simulink model "hw_ekf_est_all_para"  (R2021b)
settings: Solver=ode1  StartTime=0.0  StopTime=120  FixedStep=0.01  RelTol=1e-3  EnableMultiTasking=on
libraries: arduinolib x6, arduinosensorlib x1
settings Model: ExtModeTrigDuration=2  Creator=Admin  LastModifiedBy=ASUS
settings SolverCC: AlgebraicLoopSolver=TrustRegion  AutoInsertRateTranBlk=on
settings OptimizationCC: EnhancedBackFolding=on  PassReuseOutputArgsAs=Individual arguments  ZeroExternalMemoryAtStartup=off  ZeroInternalMemoryAtStartup=off  MaxStackSize=64  OptimizeBlockOrder=speed  DifferentSizesBufferReuse=on  OptimizationCustomize=off  EfficientTunableParamExpr=on
settings DebuggingCC: ParameterTunabilityLossMsg=error  SFMachineParentedDataDiag=warning
settings HardwareCC: ProdBitPerInt=16  ProdBitPerPointer=16  ProdBitPerSizeT=16  ProdBitPerPtrDiffT=16  ProdLargestAtomicFloat=None  ProdWordSize=8  ProdHWDeviceType=Atmel->AVR
settings SFSimCC: MATLABDynamicMemAlloc=off
settings RTWCC: Description=Embedded Coder  SystemTargetFile=ert.tlc  HardwareBoard=Arduino Mega 2560  TemplateMakefile=ert_default_tmf  Toolchain=Arduino AVR  BuildConfiguration=Faster Runs
settings CodeAppCC: ForceParamTrailComments=on  IgnoreCustomStorageClasses=off  OperatorAnnotations=on  SimulinkDataObjDesc=on  SFDataObjDesc=on  InsertBlockDesc=on
settings ERTTargetCC: SupportContinuousTime=on  SupportVariableSizeSignals=on  ExtModeTransport=3  ExtModeStaticAlloc=on  ExtModeStaticAllocSize=2048  ExtModeMexFile=ext_xcp  ExtModeIntrfLevel=Level2 - Open

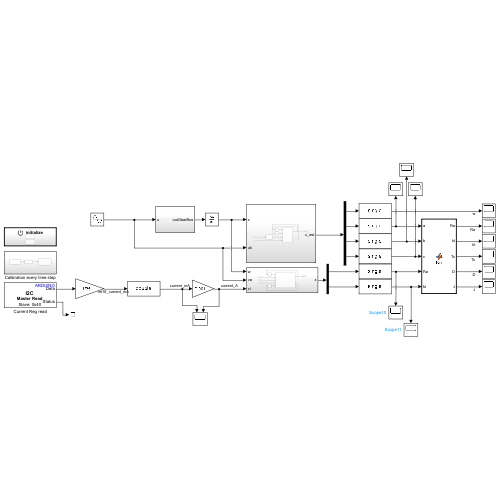
[thumbnail: Simulink's stored preview of the top-level diagram]
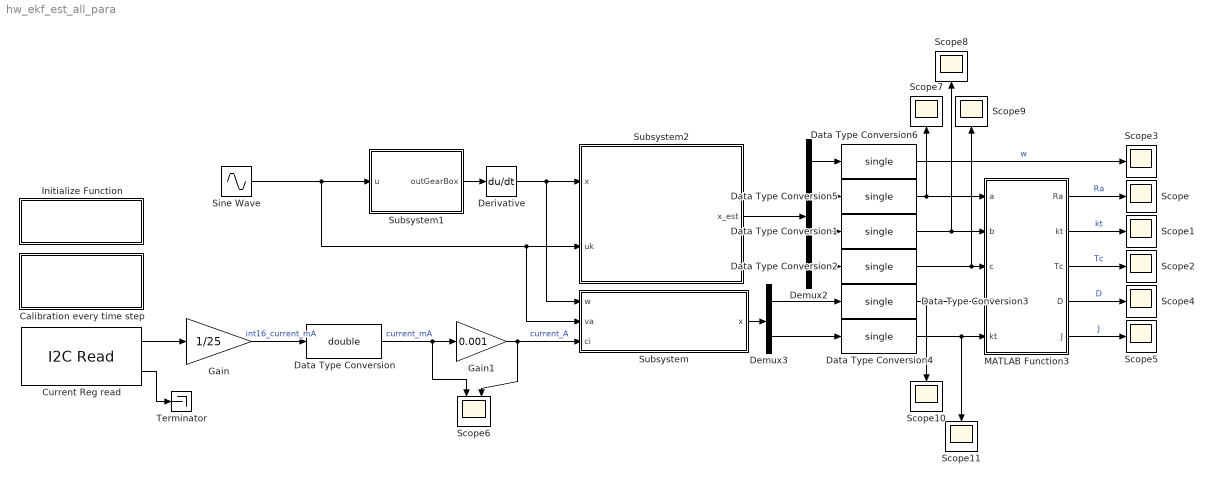
== system hw_ekf_est_all_para ==
  Calibration every time step : Subsystem  Priority=0
  Current Reg read : arduinolib/I2C Read  I2CModule=0  Mode=Master  SlaveAddress="hex2dec(\"0x40\")"  SlaveByteOrder=BigEndian  Direction=Receiver  RegisterAddressMode=on  RegisterAddress="hex2dec(\"0x04\")"  SlaveDataType=int16  DataLength=1  NoAck=off  RepeatedStart=off  OutputStatus=on  blockPlatform=ARDUINO  SampleTime=0.01
      settings: SourceProductBaseCode=ARDUINO
  Data Type Conversion : DataTypeConversion  OutDataTypeStr=double
  Data Type Conversion{1..6} (6 alike) : DataTypeConversion  OutDataTypeStr=single
  Demux2 : Demux
  Demux3 : Demux  Outputs=2
  Derivative : Derivative
  Gain : Gain  Gain=1/25
  Gain1 : Gain  Gain=0.001
  Initialize Function : Subsystem  TreatAsAtomicUnit=on
  MATLAB Function3 : MATLAB Function  TreatAsAtomicUnit=on
  Scope{,1..5,7..11} (11 alike) : Scope
  Scope6 : Scope  NumInputPorts=2
  Sine Wave : Sin  Amplitude=10  Frequency=2*pi*0.4  SampleTime=0
  Subsystem : Subsystem
  Subsystem1 : Subsystem
  Subsystem2 : Subsystem
  Terminator : Terminator
  wires:
  Demux3/2 -> Data Type Conversion4/1
  Demux2/4 -> Data Type Conversion2/1
  Demux2/3 -> Data Type Conversion1/1
  Subsystem2/1(x_est) -> Demux2/1
  Demux2/2 -> Data Type Conversion5/1
  Demux3/1 -> Data Type Conversion3/1
  Subsystem/1(x) -> Demux3/1
  Data Type Conversion/1 -> Scope6/1, Gain1/1  "current_mA"
  Current Reg read/2 -> Terminator/1
  Gain/1 -> Data Type Conversion/1  "int16_current_mA"
  Current Reg read/1 -> Gain/1
  Sine Wave/1 -> Subsystem1/1(u), Subsystem/2(va), Subsystem2/2(uk)
  Gain1/1 -> Subsystem/3(ci), Scope6/2  "current_A"
  Subsystem1/1(outGearBox) -> Derivative/1
  Derivative/1 -> Subsystem/1(w), Subsystem2/1(x)
  MATLAB Function3/1(Ra) -> Scope/1  "Ra"
  MATLAB Function3/2(kt) -> Scope1/1  "kt"
  MATLAB Function3/3(Tc) -> Scope2/1  "Tc"
  MATLAB Function3/4(D) -> Scope4/1  "D"
  MATLAB Function3/5(J) -> Scope5/1  "J"
  Demux2/1 -> Data Type Conversion6/1
  Data Type Conversion5/1 -> MATLAB Function3/1(a), Scope7/1
  Data Type Conversion1/1 -> Scope8/1, MATLAB Function3/2(b)
  Data Type Conversion2/1 -> Scope9/1, MATLAB Function3/3(c)
  Data Type Conversion3/1 -> Scope10/1, MATLAB Function3/4("Ra ")
  Data Type Conversion4/1 -> Scope11/1, MATLAB Function3/5("kt ")
  Data Type Conversion6/1 -> Scope3/1  "w"

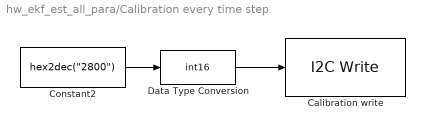
== system hw_ekf_est_all_para/Calibration every time step ==
  Calibration write : arduinolib/I2C Write  I2CModule=0  Mode=Master  SlaveAddress="uint8(hex2dec(\"0x40\"))"  SlaveByteOrder=BigEndian  Direction=Transmitter  RegisterAddressMode=on  RegisterAddress="uint8(hex2dec(\"0x05\"))"  SlaveDataType=uint8  DataLength=1  NoAck=off  RepeatedStart=off  OutputStatus=off  blockPlatform=ARDUINO
      settings: SourceProductBaseCode=ARDUINO
  Constant2 : Constant  Value="hex2dec(\"2800\")"
  Data Type Conversion : DataTypeConversion  OutDataTypeStr=int16
  wires:
  Constant2/1 -> Data Type Conversion/1
  Data Type Conversion/1 -> Calibration write/1

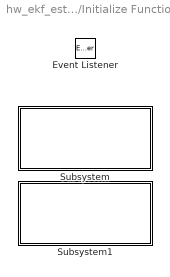
== system hw_ekf_est_all_para/Initialize Function ==
  Event Listener : EventListener  DisableCoverage=on  EventName=reset
  Subsystem : Subsystem  Priority=0
  Subsystem1 : Subsystem  Priority=1

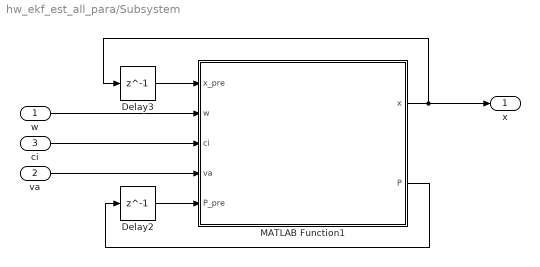
== system hw_ekf_est_all_para/Subsystem ==
  w : Inport
  va : Inport  Port=2
  ci : Inport  Port=3
  Delay2 : Delay  DelayLength=1  InitialCondition=diag([5,0.1])
  Delay3 : Delay  DelayLength=1  InitialCondition=[5;0.4]
  MATLAB Function1 : MATLAB Function  TreatAsAtomicUnit=on
  x : Outport
  wires:
  MATLAB Function1/1(x) -> x/1, Delay3/1
  Delay2/1 -> MATLAB Function1/5(P_pre)
  MATLAB Function1/2(P) -> Delay2/1
  Delay3/1 -> MATLAB Function1/1(x_pre)
  ci/1 -> MATLAB Function1/3(ci)
  w/1 -> MATLAB Function1/2(w)
  va/1 -> MATLAB Function1/4(va)

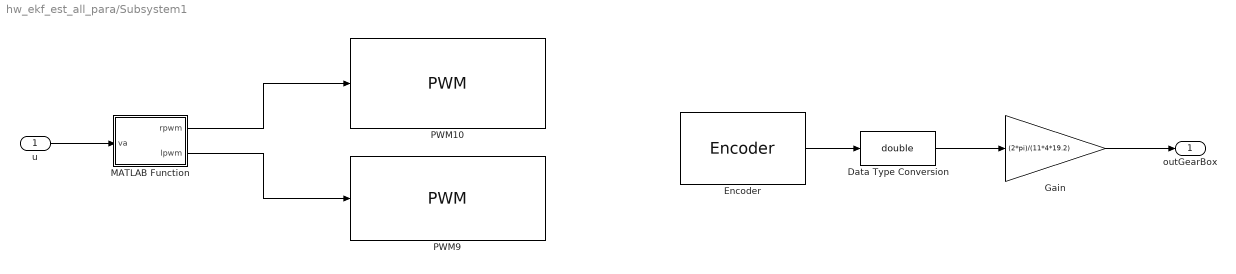
== system hw_ekf_est_all_para/Subsystem1 ==
  u : Inport
  Data Type Conversion : DataTypeConversion  OutDataTypeStr=double
  Encoder : arduinosensorlib/Encoder  InputA=2  InputB=3  Mode=No reset  SampleTime=-1
      settings: SourceProductBaseCode=ARDUINO
  Gain : Gain  Gain=(2*pi)/(11*4*19.2)
  MATLAB Function : MATLAB Function  TreatAsAtomicUnit=on
  PWM10 : arduinolib/PWM  pinNumber=8  frequencyType=Default  desiredFrequency=490.2  achievableFrequency=490.2
  PWM9 : arduinolib/PWM  pinNumber=9  frequencyType=Default  desiredFrequency=490.2  achievableFrequency=490.2
  outGearBox : Outport
  wires:
  MATLAB Function/2(lpwm) -> PWM9/1
  MATLAB Function/1(rpwm) -> PWM10/1
  u/1 -> MATLAB Function/1(va)
  Encoder/1 -> Data Type Conversion/1
  Gain/1 -> outGearBox/1
  Data Type Conversion/1 -> Gain/1

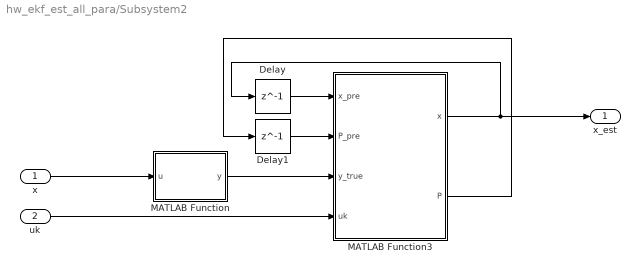
== system hw_ekf_est_all_para/Subsystem2 ==
  x : Inport
  uk : Inport  Port=2
  Delay : Delay  DelayLength=1  InitialCondition=[0;0;0;0]
  Delay1 : Delay  DelayLength=1  InitialCondition=1e0*diag([10,1,30,10])
  MATLAB Function : MATLAB Function  TreatAsAtomicUnit=on
  MATLAB Function3 : MATLAB Function  TreatAsAtomicUnit=on
  x_est : Outport
  wires:
  x/1 -> MATLAB Function/1(u)
  Delay/1 -> MATLAB Function3/1(x_pre)
  Delay1/1 -> MATLAB Function3/2(P_pre)
  MATLAB Function3/2(P) -> Delay1/1
  uk/1 -> MATLAB Function3/4(uk)
  MATLAB Function3/1(x) -> Delay/1, x_est/1
  MATLAB Function/1(y) -> MATLAB Function3/3(y_true)

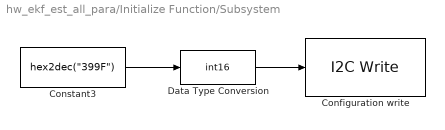
== system hw_ekf_est_all_para/Initialize Function/Subsystem ==
  Configuration write : arduinolib/I2C Write  I2CModule=0  Mode=Master  SlaveAddress="hex2dec(\"0x40\")"  SlaveByteOrder=BigEndian  Direction=Transmitter  RegisterAddressMode=on  RegisterAddress="hex2dec(\"0x00\")"  SlaveDataType=uint8  DataLength=1  NoAck=off  RepeatedStart=off  OutputStatus=off  blockPlatform=ARDUINO
      settings: SourceProductBaseCode=ARDUINO
  Constant3 : Constant  Value="hex2dec(\"399F\")"
  Data Type Conversion : DataTypeConversion  OutDataTypeStr=int16
  wires:
  Constant3/1 -> Data Type Conversion/1
  Data Type Conversion/1 -> Configuration write/1

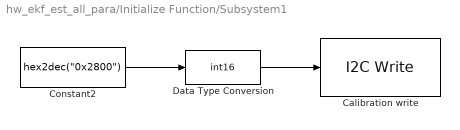
== system hw_ekf_est_all_para/Initialize Function/Subsystem1 ==
  Calibration write : arduinolib/I2C Write  I2CModule=0  Mode=Master  SlaveAddress="uint8(hex2dec(\"0x40\"))"  SlaveByteOrder=BigEndian  Direction=Transmitter  RegisterAddressMode=on  RegisterAddress="uint8(hex2dec(\"0x05\"))"  SlaveDataType=uint8  DataLength=1  NoAck=off  RepeatedStart=off  OutputStatus=off  blockPlatform=ARDUINO
      settings: SourceProductBaseCode=ARDUINO
  Constant2 : Constant  Value="hex2dec(\"0x2800\")"
  Data Type Conversion : DataTypeConversion  OutDataTypeStr=int16
  wires:
  Constant2/1 -> Data Type Conversion/1
  Data Type Conversion/1 -> Calibration write/1

== matlab function hw_ekf_est_all_para/Subsystem1/MATLAB Function ==
  data: va input; rpwm output; lpwm output
function [rpwm,lpwm] = fcn(va)

pwm = (va/24)*254;

if pwm > 0
    rpwm = pwm;
    lpwm = 0;
elseif pwm<0
    rpwm = 0;
    lpwm = abs(pwm);
else
    rpwm = 0;
    lpwm = 0;
end

== matlab function hw_ekf_est_all_para/Subsystem/MATLAB Function1 ==
  data: x_pre input; w input; ci input; va input; P_pre input; x output; P output
function [x,P] = fcn(x_pre,w,ci,va,P_pre)
% Initialize step, putted in the delay instead
% P = (A'A)^-1;
% x = P*(A'b);

% calculate state
A = [1 (w/ci)];

% recursive least square method
P = P_pre - P_pre*A'/(1+A*P_pre*A')*(A*P_pre);
K = P*A';
x = x_pre + K*((va/ci)-A*x_pre);

== matlab function hw_ekf_est_all_para/Subsystem2/MATLAB Function ==
  data: u input; y output
function y = fcn(u)

y = u(1);

== matlab function hw_ekf_est_all_para/Subsystem2/MATLAB Function3 ==
  settings: updateMethod=DISCRETE
  data: x_pre input; P_pre input; y_true input; x output; uk input; P output
function [x,P] = ekf(x_pre,P_pre,y_true, uk)
Ts = 0.01;

Qc_est  = 1e-4*diag([1,10,100,10]);
Qd_est  = Ts*Qc_est;
R_est   = 0.01;

Ck = [1 0 0 0];
Dk = 0;


% PREDICTION STEP
%Compute prediction at next time step
x = x_pre+Ts*[-x_pre(2)*x_pre(1) + uk*x_pre(3) - x_pre(4)*sign(x_pre(1));
                0;
                0;
                0];

Ak = eye(4)+Ts*[-x_pre(2) -x_pre(1) uk -sign(x_pre(1));
                 0     0    0      0;
                 0     0    0      0;
                 0     0    0      0];
P = Ak*P_pre*Ak'+Qd_est;

% OBSERVATION AND UPDATE
%Comput Kalman Gain and update predicted value
Wk    = P*Ck'/(Ck*P*Ck'+R_est);
y_est = Ck*x+Dk*uk;
dely = y_true-y_est;
Wkdely = Wk*dely;
x = x+Wkdely;
P = P-Wk*Ck*P;

== matlab function hw_ekf_est_all_para/MATLAB Function3 ==
  data: Ra output; kt output; Tc output; D output; a input; b input; c input; Ra input; J output; kt input
function [Ra,kt,Tc, D, J] = fcn(a, b, c, Ra, kt)
Ra = Ra;
kt = kt;

J = (kt/(Ra*b));
Tc = (c*J);
D = (a*Ra*J - kt^2)/Ra;
